simulink library "Lib_PF_ActiveConvEffDC2DC_TMATS"  (R2018a)
settings: Solver=ode45  StartTime=0.0  StopTime=10.0  RelTol=1e-3  EnableMultiTasking=on
Description:
  | Thomas Modules
settings Model: Creator=jwchapm2  LastModifiedBy=mebell
settings DataIOCC: LimitDataPoints=on  SaveFormat=Array
settings OptimizationCC: ExpressionDepthLimit=2147483647  LifeSpan=inf
settings DebuggingCC: UnderspecifiedInitializationDetection=Classic  MergeDetectMultiDrivingBlocksExec=none  SolverPrmCheckMsg=warning  StateNameClashWarn=warning  SFUnexpectedBacktrackingDiag=warning  SFNoUnconditionalDefaultTransitionDiag=warning  SFExecutionAtInitializationDiag=none
settings HardwareCC: ProdBitPerPointer=32  ProdBitPerSizeT=32  ProdBitPerPtrDiffT=32  ProdLargestAtomicFloat=None  ProdIntDivRoundTo=Undefined  ProdEndianess=Unspecified  ProdWordSize=32  ProdHWDeviceType=32-bit Generic
settings ModelReferenceCC: PropagateSignalLabelsOutOfModel=off
settings CodeAppCC: StateflowObjectComments=on
settings GRTTargetCC: TargetLangStandard=C89/C90 (ANSI)  GeneratePreprocessorConditionals=Disable all
settings ConfigComp: CovMetricSettings=dw  CovHtmlReporting=on  CovSaveCumulativeToWorkspaceVar=on  CovSaveSingleToWorkspaceVar=on  CovExternalEMLEnable=off

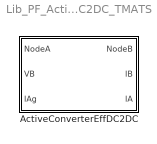
== system Lib_PF_ActiveConvEffDC2DC_TMATS ==
  ActiveConverterEffDC2DC : Subsystem  mask{EffInEN_M=off, Eff_M=98, BlkNm_M=double(gcb)}
      mask prompts: EffInEN_M "EffInEN_M - Externally Defined Efficiency"; Eff_M "Eff_M - Converter Efficiency"; BlkNm_M "Block name as double for simulink output"
      mask init:
      | %Manage Inputs
      | if EffInEN_M == 1
      |     if strcmp(get_param([BlkNm_M '/Eff'],'BlockType'),'Constant')
      |         MSK_ReplaceBlock_TMATS([BlkNm_M '/Eff'],'built-in/Inport');
      |     end
      |     set_param([BlkNm_M '/Eff'],'Port',num2str(4));
      | elseif EffInEN_M == 0
      |     if strcmp(get_param([BlkNm_M '/Eff'],'BlockType'),'Inport')
      |         MSK_ReplaceBlock_TMATS([BlkNm_M '/Eff'],'built-in/Constant');
      |         set_param([BlkNm_M '/Eff'],'Value','Eff_M');
      |     end
      | end
      mask Callback EffInEN_M: MSK_SEC_Enables_TMATS('EffInEN_M',2,'dis')
      mask Display:
      | fprintf('DC : DC')
      | port_label('input',1,'VA')
      | port_label('input',2,'VB')
      | port_label('input',3,'IAg')
      | if EffInEN_M == 1
      | port_label('input',4,'Eff')
      | end
      | port_label('output',1,'VB')
      | port_label('output',2,'IB')
      | port_label('output',3,'IA')

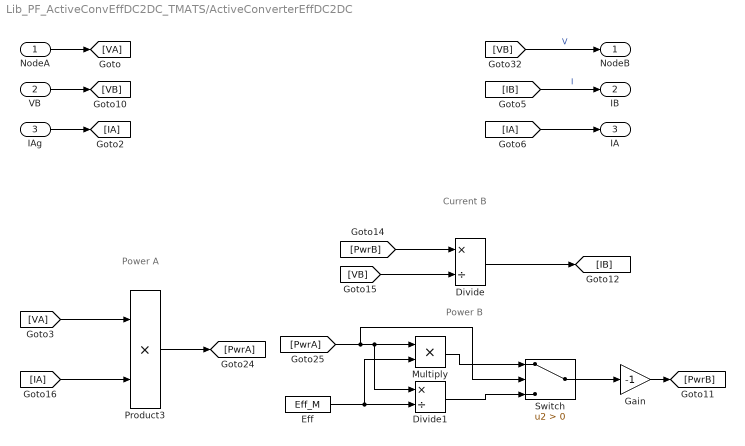
== system Lib_PF_ActiveConvEffDC2DC_TMATS/ActiveConverterEffDC2DC ==
  note: Power A
  note: Current B
  note: Power B
  NodeA : Inport
  VB : Inport  Port=2
  IAg : Inport  Port=3
  Divide : Product  Inputs=*/
  Divide1 : Product  Inputs=*/
  Eff : Constant  Value=Eff_M
  Gain : Gain  Gain=-1
  Multiply : Product
  Product3 : Product
  Switch : Switch  Criteria=u2 > Threshold
  NodeB : Outport
  IB : Outport  Port=2
  IA : Outport  Port=3
  wires:
  [VA] -> Product3/1
  Product3/1 -> [PwrA]
  [VB] -> NodeB/1  "V"
  NodeA/1 -> [VA]
  [IA] -> Product3/2
  Gain/1 -> [PwrB]
  [PwrB] -> Divide/1
  Switch/1 -> Gain/1
  [PwrA] -> Switch/2, Divide1/1, Multiply/1
  Divide/1 -> [IB]
  [VB] -> Divide/2
  IAg/1 -> [IA]
  [IB] -> IB/1  "I"
  Eff/1 -> Multiply/2, Divide1/2
  VB/1 -> [VB]
  [IA] -> IA/1
  Divide1/1 -> Switch/3
  Multiply/1 -> Switch/1
